simulink model "out_double_UnitDelay"  (R2014a)
settings: Solver=FixedStepDiscrete  StartTime=0.0  StopTime=10.0  FixedStep=0.1  RelTol=1e-3
settings Model: Creator=yoshi12  LastModifiedBy=yoshi12

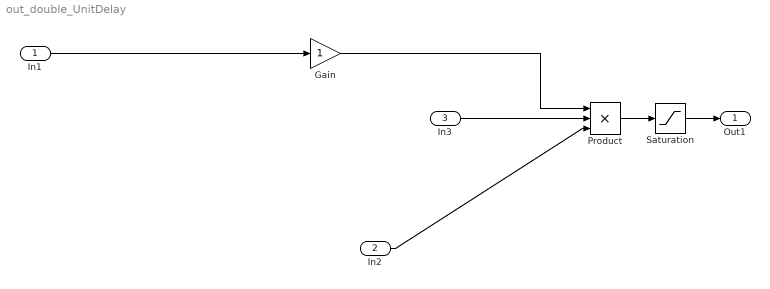
== system out_double_UnitDelay ==
  In1 : Inport
  In2 : Inport  Port=2
  In3 : Inport  Port=3
  Gain : Gain
  Product : Product  Inputs=3
  Saturation : Saturate
  Out1 : Outport
  wires:
  In1/1 -> Gain/1
  Gain/1 -> Product/1
  Product/1 -> Saturation/1
  Saturation/1 -> Out1/1
  In2/1 -> Product/3
  In3/1 -> Product/2
